simulink model "Laenge_Lastheber"  (R2016b)
settings: Solver=VariableStepAuto  StartTime=0.0  StopTime=10.0  RelTol=1e-3
settings Model: Creator=nicol  LastModifiedBy=nicol

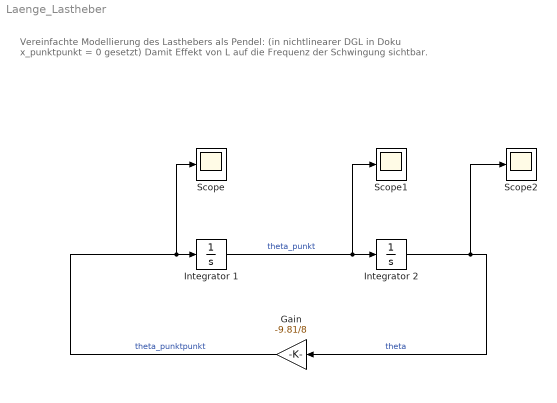
== system Laenge_Lastheber ==
  note: Vereinfachte Modellierung des Lasthebers als Pendel:
      | (in nichtlinearer DGL in Doku x_punktpunkt = 0 gesetzt)
      |
      | Damit Effekt von L auf die Frequenz der Schwingung sichtbar.
  Gain : Gain  Gain=-9.81/8
  Integrator 1 : Integrator
  Integrator 2 : Integrator  InitialCondition=1
  Scope : Scope
  Scope1 : Scope
  Scope2 : Scope
  wires:
  Integrator 1/1 -> Scope1/1, Integrator 2/1  "theta_punkt"
  Integrator 2/1 -> Scope2/1, Gain/1  "theta"
  Gain/1 -> Scope/1, Integrator 1/1  "theta_punktpunkt"
